simulink model "Vin12V_Vout48V"  (R2016a)
settings: Solver=ode3  SolverMode=SingleTasking  StartTime=0.0  StopTime=0.25  FixedStep=1e-6  MaxStep=1e-4  RelTol=1e-4
libraries: powerlib x13, simulink x1
settings Model: Creator=A0109971  LastModifiedBy=Qosmıo
settings DataIOCC: SaveFormat=StructureWithTime
settings DebuggingCC: SFUnexpectedBacktrackingDiag=error  SFNoUnconditionalDefaultTransitionDiag=error
settings HardwareCC: ProdWordSize=32  ProdHWDeviceType=Specified
settings GRTTargetCC: TargetLangStandard=C99 (ISO)  GeneratePreprocessorConditionals=Use local settings
settings ConfigComp: CovMetricSettings=dwe  CovHtmlReporting=off  CovSaveCumulativeToWorkspaceVar=off  CovSaveSingleToWorkspaceVar=off  CovModelRefEnable=Off  CovExternalEMLEnable=on

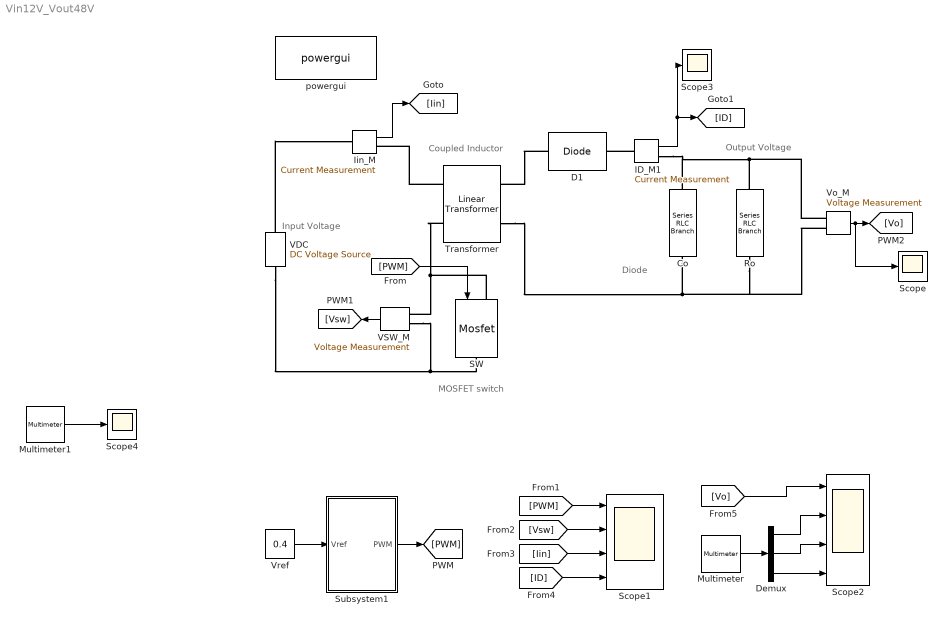
== system Vin12V_Vout48V ==
  note: Coupled Inductor
  note: Input Voltage
  note: MOSFET switch
  note: Diode
  note: Output Voltage
  Co : powerlib/Elements/Series RLC Branch  LConnTagsString=__new0  RConnTagsString=__new0  BranchType=C  Resistance=1  Inductance=1e-3  SetiL0=off  InitialCurrent=0  Capacitance=100e-6  Setx0=off  InitialVoltage=0  Measurements=None
  D1 : powerlib/Power Electronics/Diode  Ron=0.001  Lon=0  Vf=0.8  IC=0  UseSnubber=off  Rs=500*inf  Cs=250e-9  Measurements=off
  Demux : Demux  Outputs=3
  ID_M1 : powerlib/Measurements/Current Measurement  PhasorSimulation=off  OutputType=Complex  PSBequivalent=0
  Iin_M : powerlib/Measurements/Current Measurement  PhasorSimulation=off  OutputType=Complex  PSBequivalent=0
  Multimeter : powerlib/Measurements/Multimeter  PhasorSimulation=off  OutputType=Complex  sel=[3 7 1]  L=8  Gain=[1 1 1]  yselected={'Ib: Ro','Imag: Transformer','Uw1: Transformer'};  PSBOutputType=1  PSBequivalent=0  AxesSetting=[0,0.1,-100,100]  Display=0  SavedBlockNames=-11
  Multimeter1 : powerlib/Measurements/Multimeter  PhasorSimulation=off  OutputType=Complex  sel=7  L=8  Gain=1  yselected={'Imag: Transformer'};  PSBOutputType=1  PSBequivalent=0  AxesSetting=[0,0.1,-100,100]  Display=0  SavedBlockNames=-11
  Ro : powerlib/Elements/Series RLC Branch  LConnTagsString=__new0  RConnTagsString=__new0  BranchType=R  Resistance=25.6  Inductance=1e-3  SetiL0=off  InitialCurrent=0  Capacitance=1e-6  Setx0=off  InitialVoltage=0  Measurements=Branch current
  SW : powerlib/Power Electronics/Mosfet  Ron=0.1  Lon=0  Rd=0.01  Vfd=0  IC=0  Rs=1e5  Cs=inf  Measurements=off
  Scope : Scope
  Scope1 : Scope  NumInputPorts=4
  Scope2 : Scope  NumInputPorts=4
  Scope3 : Scope
  Scope4 : Scope
  Subsystem1 : Subsystem
  Transformer : powerlib/Elements/Linear Transformer  UNITS=SI  NominalPower=[ 1000 100e3 ]  winding1=[500 0 0]  winding2=[3000 0 0]  ThreeWindings=off  winding3=[3.15e+05 315.06 8.8673e-08]  RmLm=[1 75e-6]  Measurements=All voltages and currents  DataType=on
  VDC : powerlib/Electrical Sources/DC Voltage Source  Amplitude=12  Measurements=None
  VSW_M : powerlib/Measurements/Voltage Measurement  PhasorSimulation=off  OutputType=Complex  PSBequivalent=0
  Vo_M : powerlib/Measurements/Voltage Measurement  PhasorSimulation=off  OutputType=Complex  PSBequivalent=0
  Vref : Constant  Value=0.4
  powergui : powerlib/powergui  Priority=1  SimulationMode=Continuous  SolverType=Tustin/Backward Euler (TBE)  SampleTime=1e-6  frequency=60  SPID=on  DisableSnubberDevices=off  DisableRonSwitches=off  DisableVfSwitches=off  SwTol=0  DisplayEquations=off  Interpol=off  ExternalGateDelay=off  methode=off  Ts=100  FunctionMessages=off  echomessages=off  HookPort=off  EnableUseOfTLC=off  x0status=blocks  frequencyindice=0  Pbase=100e6  ErrMax=1e-4  Iterations=50  UnitsV=kV  UnitsW=MW  buscounter=0  RestoreLinks=warning  ResistiveCurrentMeasurement=off  Frange=[0:2:500]  Ylog=off  Xlog=on  ShowGrid=off  save=off  variable=ZData  structure=0  ZoomFFT=off  StartTime=0.0  cycles=1  DisplayStyle=1  fundamental=60  FreqAxis=off  MaxFrequency=1000  frequencyindicesteady=1  RmsSteady=1  display=off
  wires:
  [PWM] -> SW/1
  [PWM] -> Scope1/1
  VSW_M/1 -> [Vsw]
  [Vsw] -> Scope1/2
  Iin_M/1 -> [Iin]
  [Iin] -> Scope1/3
  Vo_M/1 -> Scope/1, [Vo]
  [ID] -> Scope1/4
  [Vo] -> Scope2/1
  Demux/2 -> Scope2/3
  Demux/1 -> Scope2/2
  Demux/3 -> Scope2/4
  Multimeter/1 -> Demux/1
  Vref/1 -> Subsystem1/1(Vref)
  Subsystem1/1("PWM ") -> [PWM]
  ID_M1/1 -> Scope3/1, [ID]
  Multimeter1/1 -> Scope4/1
  connections:
  SW/LConn1 -- Transformer/LConn2 -- VSW_M/LConn1
  VDC/LConn1 -- VSW_M/LConn2 -- SW/RConn1
  Ro/RConn1 -- Co/RConn1 -- ID_M1/RConn1 -- Vo_M/LConn2
  VDC/RConn1 -- Iin_M/LConn1
  Vo_M/LConn1 -- Ro/LConn1 -- Co/LConn1 -- Transformer/RConn2
  Transformer/LConn1 -- Iin_M/RConn1
  D1/LConn1 -- Transformer/RConn1
  ID_M1/LConn1 -- D1/RConn1

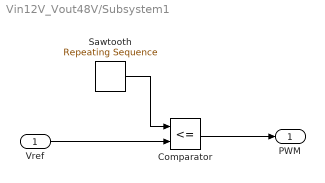
== system Vin12V_Vout48V/Subsystem1 ==
  Vref : Inport
  Comparator : RelationalOperator  Operator=<=  OutDataTypeStr=boolean
  Sawtooth : simulink/Sources/Repeating Sequence  rep_seq_t=[0 1e-4]  rep_seq_y=[0 1]
  "PWM " : Outport
  wires:
  Sawtooth/1 -> Comparator/1
  Vref/1 -> Comparator/2
  Comparator/1 -> "PWM "/1
